simulink model "Vehicle_Motion_Model_R2014a"  (R2014a)
settings: Solver=ode4  SolverMode=SingleTasking  StartTime=0.0  StopTime=10.0  FixedStep=0.001  RelTol=1e-3
values from neighbouring files (symbols this model uses):
  chassis_real = chassis    [Parameters_Chassis.m]
  mu = [1 1 1 1]    [Parameters_Initialization.m]
  psi0 = 0    [Parameters_Initialization.m]
  psip0 = 0    [Parameters_Initialization.m]
  vx0 = 15    [Parameters_Initialization.m]
  vy0 = 0    [Parameters_Initialization.m]
  x0 = 0    [Parameters_Initialization.m]
  y0 = 0    [Parameters_Initialization.m]
undefined symbols (not defined in the file or in its folder): DiscIntNeverNeededParam, tireparam
libraries: vrlib x6, simulink x2
settings Model: CovMetricSettings=dwe  CovHtmlReporting=off  covSaveCumulativeToWorkspaceVar=off  CovSaveSingleToWorkspaceVar=off  CovExternalEMLEnable=on  CovSFcnEnable=on  Creator=Leo  LastModifiedBy=Leo
settings DataIOCC: LimitDataPoints=off  SaveFormat=StructureWithTime
settings DebuggingCC: MergeDetectMultiDrivingBlocksExec=error  SolverPrmCheckMsg=none  FrameProcessingCompatibilityMsg=error  SFUnexpectedBacktrackingDiag=error  SFNoUnconditionalDefaultTransitionDiag=error
settings HardwareCC: ProdBitPerPointer=64  ProdLargestAtomicFloat=Float  ProdIntDivRoundTo=Zero  ProdEndianess=LittleEndian  ProdHWDeviceType=Specified
settings ModelReferenceCC: PropagateSignalLabelsOutOfModel=on
settings GRTTargetCC: TargetLangStandard=C99 (ISO)  GeneratePreprocessorConditionals=Use local settings

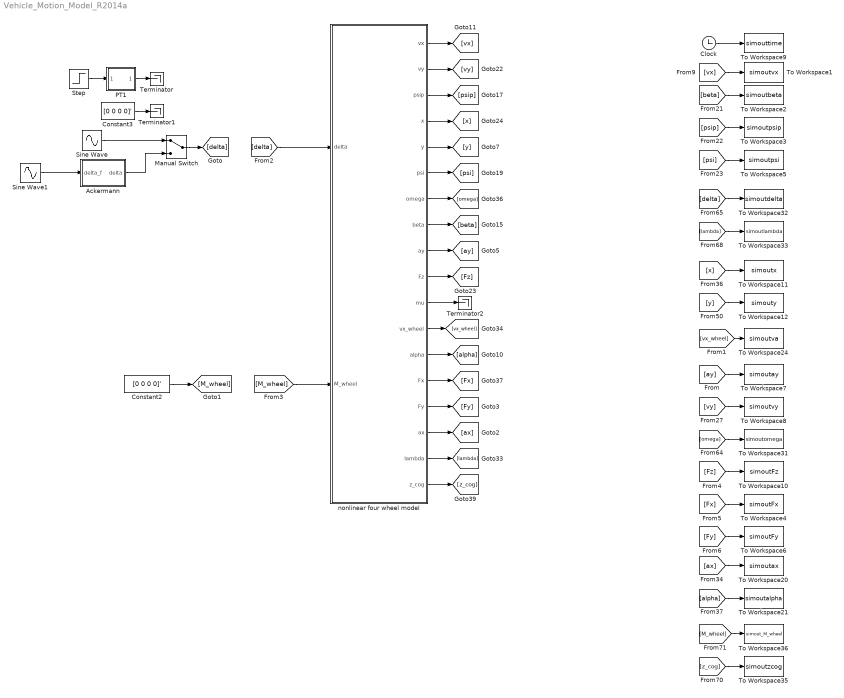
== system Vehicle_Motion_Model_R2014a ==
  Ackermann : Subsystem
  Clock : Clock
  Constant2 : Constant  Value=[0 0 0 0]'
  Constant3 : Constant  Value=[0 0 0 0]'
  Manual Switch : ManualSwitch
  PT1 : Subsystem
  Sine Wave : Sin  Amplitude=30/180*pi*[1 1 0 0]  Frequency=3  SampleTime=0
  Sine Wave1 : Sin  Amplitude=30/180*pi  Frequency=3  SampleTime=0
  Step : Step  Time=0.5  After=30/180*pi*[1 1 0 0]  SampleTime=0
  Terminator : Terminator
  Terminator1 : Terminator
  Terminator2 : Terminator
  To Workspace1 : ToWorkspace  VariableName=simoutvx  SaveFormat=Timeseries  SampleTime=-1
  To Workspace10 : ToWorkspace  VariableName=simoutFz  SaveFormat=Timeseries  SampleTime=-1
  To Workspace11 : ToWorkspace  VariableName=simoutx  SaveFormat=Timeseries  SampleTime=-1
  To Workspace12 : ToWorkspace  VariableName=simouty  SaveFormat=Timeseries  SampleTime=-1
  To Workspace2 : ToWorkspace  VariableName=simoutbeta  SaveFormat=Timeseries  SampleTime=-1
  To Workspace20 : ToWorkspace  VariableName=simoutax  SaveFormat=Timeseries  SampleTime=-1
  To Workspace21 : ToWorkspace  VariableName=simoutalpha  SaveFormat=Timeseries  SampleTime=-1
  To Workspace24 : ToWorkspace  VariableName=simoutva  SaveFormat=Timeseries  SampleTime=-1
  To Workspace3 : ToWorkspace  VariableName=simoutpsip  SaveFormat=Timeseries  SampleTime=-1
  To Workspace31 : ToWorkspace  VariableName=simoutomega  SaveFormat=Timeseries  SampleTime=-1
  To Workspace32 : ToWorkspace  VariableName=simoutdelta  SaveFormat=Timeseries  SampleTime=-1
  To Workspace33 : ToWorkspace  VariableName=simoutlambda  SaveFormat=Timeseries  SampleTime=-1
  To Workspace35 : ToWorkspace  VariableName=simoutzcog  SaveFormat=Timeseries  SampleTime=-1
  To Workspace36 : ToWorkspace  VariableName=simout_M_wheel  SaveFormat=Timeseries  SampleTime=-1
  To Workspace4 : ToWorkspace  VariableName=simoutFx  SaveFormat=Timeseries  SampleTime=-1
  To Workspace5 : ToWorkspace  VariableName=simoutpsi  SaveFormat=Timeseries  SampleTime=-1
  To Workspace6 : ToWorkspace  VariableName=simoutFy  SaveFormat=Timeseries  SampleTime=-1
  To Workspace7 : ToWorkspace  VariableName=simoutay  SaveFormat=Timeseries  SampleTime=-1
  To Workspace8 : ToWorkspace  VariableName=simoutvy  SaveFormat=Timeseries  SampleTime=-1
  To Workspace9 : ToWorkspace  VariableName=simouttime  SampleTime=-1
  nonlinear four wheel model : Subsystem  Description=|
      | vereinfachte alpha
      | beta=vs/vl
  wires:
  Step/1 -> PT1/1(In1)
  [delta] -> nonlinear four wheel model/1(delta)
  [lambda] -> To Workspace33/1
  [beta] -> To Workspace2/1
  [vx_wheel] -> To Workspace24/1
  nonlinear four wheel model/9(ay) -> [ay]
  [M_wheel] -> To Workspace36/1
  [z_cog] -> To Workspace35/1
  [delta] -> To Workspace32/1
  nonlinear four wheel model/10(Fz) -> [Fz]
  nonlinear four wheel model/12(vx_wheel) -> [vx_wheel]
  [y] -> To Workspace12/1
  [omega] -> To Workspace31/1
  [vy] -> To Workspace8/1
  [alpha] -> To Workspace21/1
  Clock/1 -> To Workspace9/1
  [ax] -> To Workspace20/1
  nonlinear four wheel model/14(Fx) -> [Fx]
  Sine Wave1/1 -> Ackermann/1(delta_f)
  [vx] -> To Workspace1/1
  [x] -> To Workspace11/1
  nonlinear four wheel model/6(psi) -> [psi]
  nonlinear four wheel model/16(ax) -> [ax]
  nonlinear four wheel model/5(y) -> [y]
  [psip] -> To Workspace3/1
  nonlinear four wheel model/7(omega) -> [omega]
  nonlinear four wheel model/11(mu) -> Terminator2/1
  nonlinear four wheel model/13(alpha) -> [alpha]
  nonlinear four wheel model/1(vx) -> [vx]
  nonlinear four wheel model/18(z_cog) -> [z_cog]
  [ay] -> To Workspace7/1
  nonlinear four wheel model/2(vy) -> [vy]
  [psi] -> To Workspace5/1
  nonlinear four wheel model/3(psip) -> [psip]
  nonlinear four wheel model/17(lambda) -> [lambda]
  [M_wheel] -> nonlinear four wheel model/2(M_wheel)
  nonlinear four wheel model/4(x) -> [x]
  nonlinear four wheel model/8(beta) -> [beta]
  Sine Wave/1 -> Manual Switch/1
  Ackermann/1(delta) -> Manual Switch/2
  PT1/1(Out1) -> Terminator/1
  Constant3/1 -> Terminator1/1
  Manual Switch/1 -> [delta]
  Constant2/1 -> [M_wheel]
  [Fy] -> To Workspace6/1
  [Fx] -> To Workspace4/1
  [Fz] -> To Workspace10/1
  nonlinear four wheel model/15(Fy) -> [Fy]

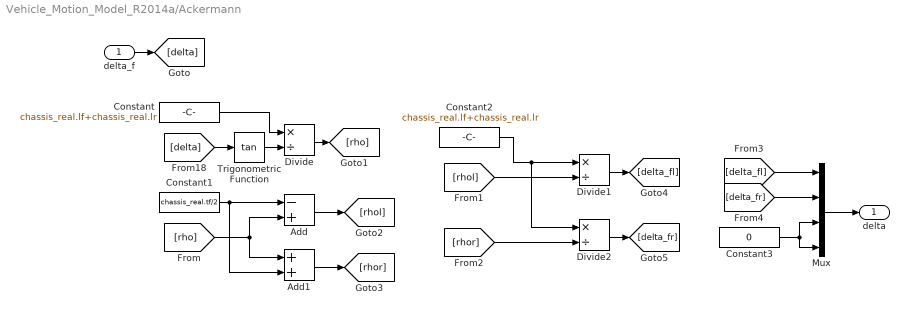
== system Vehicle_Motion_Model_R2014a/Ackermann ==
  delta_f : Inport
  Add : Sum  Inputs=-+
  Add1 : Sum
  Constant : Constant  Value=chassis_real.lf+chassis_real.lr
  Constant1 : Constant  Value=chassis_real.tf/2
  Constant2 : Constant  Value=chassis_real.lf+chassis_real.lr
  Constant3 : Constant  Value=0
  Divide : Product  Inputs=*/
  Divide1 : Product  Inputs=*/
  Divide2 : Product  Inputs=*/
  Mux : Mux
  Trigonometric Function : Trigonometry  Operator=tan
  delta : Outport
  wires:
  delta_f/1 -> [delta]
  [delta] -> Trigonometric Function/1
  Trigonometric Function/1 -> Divide/2
  Constant/1 -> Divide/1
  Divide/1 -> [rho]
  Add/1 -> [rhol]
  [rho] -> Add/2, Add1/1
  Constant1/1 -> Add1/2, Add/1
  Add1/1 -> [rhor]
  Constant2/1 -> Divide2/1, Divide1/1
  [rhol] -> Divide1/2
  [rhor] -> Divide2/2
  Divide1/1 -> [delta_fl]
  Divide2/1 -> [delta_fr]
  Mux/1 -> delta/1
  [delta_fl] -> Mux/1
  [delta_fr] -> Mux/2
  Constant3/1 -> Mux/4, Mux/3

== system Vehicle_Motion_Model_R2014a/PT1 ==
  In1 : Inport
  Add : Sum  Inputs=+-
  Gain : Gain
  Integrator : Integrator
  Out1 : Outport
  wires:
  Add/1 -> Integrator/1
  Integrator/1 -> Gain/1
  Gain/1 -> Add/2, Out1/1
  In1/1 -> Add/1

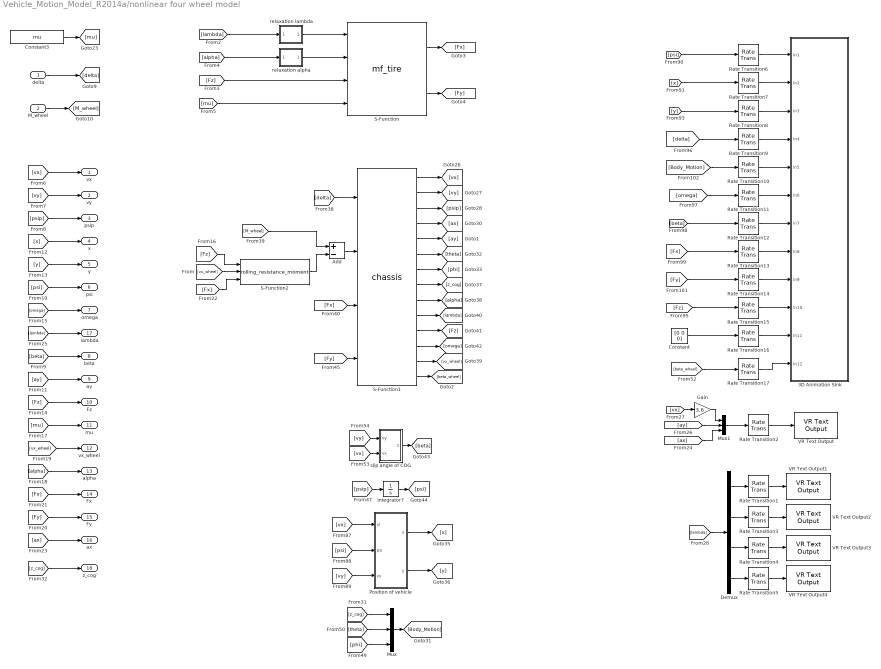
== system Vehicle_Motion_Model_R2014a/nonlinear four wheel model ==
  delta : Inport
  M_wheel : Inport  Port=2
  3D Animation Sink : Subsystem
  Add : Sum  Inputs=+-
  Constant : Constant  Value=[0 0 0]
  Constant3 : Constant  Value=mu
  Demux : Demux
  Gain : Gain  Gain=3.6
  Integrator7 : Integrator  InitialCondition=psi0
  Mux : Mux  Inputs=3
  Mux1 : Mux  Inputs=3
  Position of vehicle : Subsystem
  Rate Transition{1..17} (17 alike) : RateTransition  Integrity=off
  S-Function : S-Function  FunctionName=mf_tire  Parameters=tireparam.ov,tireparam.fxp,tireparam.fyp,tireparam.fxc,tireparam.fyc  SFunctionDeploymentMode=off  EnableBusSupport=off
  S-Function1 : S-Function  FunctionName=chassis  Parameters=chassis_real.lf,chassis_real.lr,chassis_real.tf,chassis_real.tr,chassis_real.m,chassis_real.jz,chassis_real.jy,chassis_real.jx,chassis_real.h,chassis_real.df,chassis_real.dr,chassis_real.kf,chassis_real.kr,chassis_real.jwheel,chassis_real.rwheel,vx0,vy0,psip0  SFunctionDeploymentMode=off  EnableBusSupport=off
  S-Function2 : S-Function  FunctionName=rolling_resistance_moment  Parameters=tireparam.ov,tireparam.mroll  SFunctionDeploymentMode=off  EnableBusSupport=off
  VR Text Output : vrlib/VR Text Output  VrmlFile=Virtual World Vehicle.wrl  TxtNode=lefttop  FormatString="Speed  :  %3.1f km/h \\nay        :  %1.1f g \\nax        :  %1.1f g"  Ts=0.01  ForceViewerOpen=off
  VR Text Output1 : vrlib/VR Text Output  VrmlFile=Virtual World Vehicle.wrl  TxtNode=lft  FormatString=%1.2f  Ts=0.01  ForceViewerOpen=off
  VR Text Output2 : vrlib/VR Text Output  VrmlFile=Virtual World Vehicle.wrl  TxtNode=rft  FormatString=%1.2f  Ts=0.01  ForceViewerOpen=off
  VR Text Output3 : vrlib/VR Text Output  VrmlFile=Virtual World Vehicle.wrl  TxtNode=lrt  FormatString=%1.2f  Ts=0.01  ForceViewerOpen=off
  VR Text Output4 : vrlib/VR Text Output  VrmlFile=Virtual World Vehicle.wrl  TxtNode=rrt  FormatString=%1.2f  Ts=0.01  ForceViewerOpen=off
  relaxation alpha : Subsystem
  relaxation lambda : Subsystem
  slip angle of COG : Subsystem
  vx : Outport
  vy : Outport  Port=2
  psip : Outport  Port=3
  x : Outport  Port=4
  y : Outport  Port=5
  psi : Outport  Port=6
  omega : Outport  Port=7
  beta : Outport  Port=8
  ay : Outport  Port=9
  Fz : Outport  Port=10
  mu : Outport  Port=11
  vx_wheel : Outport  Port=12
  alpha : Outport  Port=13
  Fx : Outport  Port=14
  Fy : Outport  Port=15
  ax : Outport  Port=16
  lambda : Outport  Port=17
  z_cog : Outport  Port=18
  wires:
  Constant3/1 -> [mu]
  [vx] -> Position of vehicle/1(vl)
  [psi] -> Position of vehicle/2(psi)
  [vy] -> Position of vehicle/3(vs)
  Position of vehicle/1(x) -> [x]
  Position of vehicle/2(y) -> [y]
  delta/1 -> [delta]
  [vx] -> vx/1
  [vy] -> vy/1
  [psip] -> psip/1
  [psi] -> psi/1
  [ay] -> ay/1
  [beta] -> beta/1
  [x] -> x/1
  [y] -> y/1
  [omega] -> omega/1
  [Fz] -> Fz/1
  [mu] -> mu/1
  [vx_wheel] -> vx_wheel/1
  [alpha] -> alpha/1
  [Fx] -> Fx/1
  [Fy] -> Fy/1
  [ax] -> ax/1
  [lambda] -> lambda/1
  [z_cog] -> z_cog/1
  [omega] -> Rate Transition11/1
  [delta] -> Rate Transition9/1
  [psi] -> Rate Transition6/1
  [x] -> Rate Transition7/1
  [beta] -> Rate Transition12/1
  [Fx] -> Rate Transition13/1
  [Body_Motion] -> Rate Transition10/1
  [Fy] -> Rate Transition14/1
  [y] -> Rate Transition8/1
  [Fz] -> Rate Transition15/1
  Mux/1 -> [Body_Motion]
  [phi] -> Mux/3
  [theta] -> Mux/2
  [z_cog] -> Mux/1
  Mux1/1 -> Rate Transition2/1
  [ay] -> Mux1/2
  [vx] -> Gain/1
  [ax] -> Mux1/3
  Rate Transition2/1 -> VR Text Output/1
  Rate Transition1/1 -> VR Text Output1/1
  Demux/1 -> Rate Transition1/1
  [lambda] -> Demux/1
  Rate Transition3/1 -> VR Text Output2/1
  Demux/2 -> Rate Transition3/1
  Rate Transition4/1 -> VR Text Output3/1
  Demux/3 -> Rate Transition4/1
  Rate Transition5/1 -> VR Text Output4/1
  Demux/4 -> Rate Transition5/1
  Rate Transition6/1 -> 3D Animation Sink/1(In1)
  Rate Transition7/1 -> 3D Animation Sink/2(In2)
  Rate Transition8/1 -> 3D Animation Sink/3(In3)
  Rate Transition9/1 -> 3D Animation Sink/4(In4)
  Rate Transition10/1 -> 3D Animation Sink/5(In5)
  Rate Transition11/1 -> 3D Animation Sink/6(In6)
  Rate Transition12/1 -> 3D Animation Sink/7(In7)
  Rate Transition13/1 -> 3D Animation Sink/8(In8)
  Rate Transition14/1 -> 3D Animation Sink/9(In9)
  Rate Transition15/1 -> 3D Animation Sink/10(In10)
  Gain/1 -> Mux1/1
  M_wheel/1 -> [M_wheel]
  Integrator7/1 -> [psi]
  S-Function1/7 -> [phi]
  [psip] -> Integrator7/1
  [delta] -> S-Function1/1
  S-Function1/8 -> [z_cog]
  S-Function1/5 -> [ay]
  S-Function1/4 -> [ax]
  S-Function1/1 -> [vx]
  S-Function1/11 -> [Fz]
  [Fx] -> S-Function1/3
  [Fy] -> S-Function1/4
  S-Function1/3 -> [psip]
  S-Function1/12 -> [omega]
  [M_wheel] -> Add/1
  S-Function1/10 -> [lambda]
  S-Function1/2 -> [vy]
  S-Function1/6 -> [theta]
  S-Function1/9 -> [alpha]
  S-Function1/13 -> [vx_wheel]
  Rate Transition17/1 -> 3D Animation Sink/12(In12)
  [beta_wheel] -> Rate Transition17/1
  [mu] -> S-Function/4
  [lambda] -> relaxation lambda/1(In1)
  [Fz] -> S-Function/3
  S-Function/1 -> [Fx]
  S-Function/2 -> [Fy]
  [alpha] -> relaxation alpha/1(In1)
  relaxation lambda/1(Out1) -> S-Function/1
  relaxation alpha/1(Out1) -> S-Function/2
  [vy] -> slip angle of COG/1(vy)
  [vx] -> slip angle of COG/2(vx)
  slip angle of COG/1(beta) -> [beta]
  Add/1 -> S-Function1/2
  [vx_wheel] -> S-Function2/2
  [Fz] -> S-Function2/1
  [Fx] -> S-Function2/3
  S-Function1/14 -> [beta_wheel]
  S-Function2/1 -> Add/2
  Rate Transition16/1 -> 3D Animation Sink/11(In11)
  Constant/1 -> Rate Transition16/1

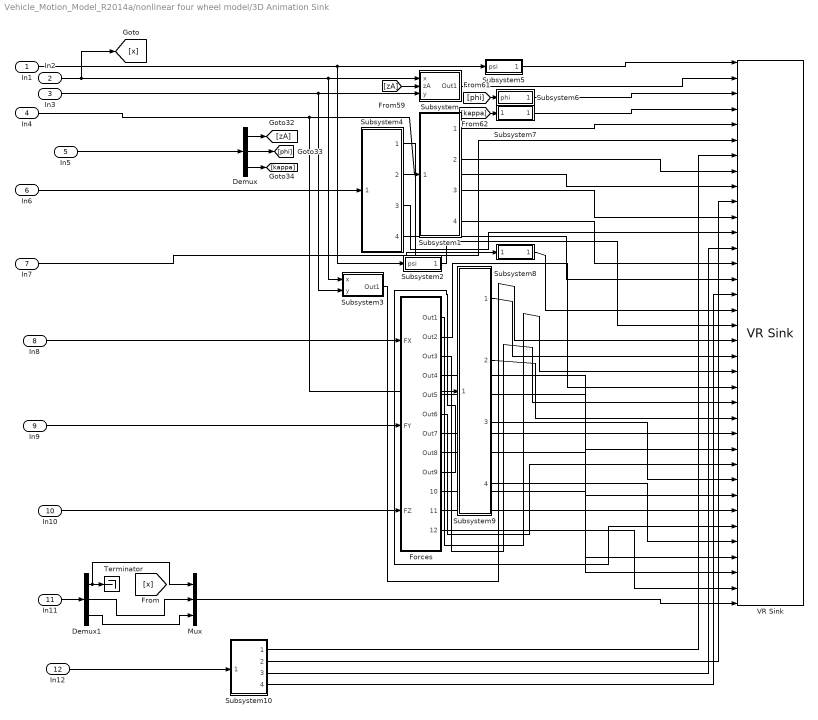
== system Vehicle_Motion_Model_R2014a/nonlinear four wheel model/3D Animation Sink ==
  In1 : Inport
  In2 : Inport  Port=2
  In3 : Inport  Port=3
  In4 : Inport  Port=4
  In5 : Inport  Port=5
  In6 : Inport  Port=6
  In7 : Inport  Port=7
  In8 : Inport  Port=8
  In9 : Inport  Port=9
  In10 : Inport  Port=10
  In11 : Inport  Port=11
  In12 : Inport  Port=12
  Demux : Demux  Outputs=3
  Demux1 : Demux  Outputs=3
  Forces : Subsystem
  Mux : Mux  Inputs=3
  Subsystem : Subsystem
  Subsystem1 : Subsystem
  Subsystem10 : Subsystem
  Subsystem2 : Subsystem
  Subsystem3 : Subsystem
  Subsystem4 : Subsystem
  Subsystem5 : Subsystem
  Subsystem6 : Subsystem
  Subsystem7 : Subsystem
  Subsystem8 : Subsystem
  Subsystem9 : Subsystem
  Terminator : Terminator
  VR Sink : vrlib/VR Sink  InstantiateOnLoad=on  SampleTime=0.02  ViewEnable=on  RemoteChange=off  RemoteView=off  FieldsWritten=Carbody.rotation.4.1.1.double#Carbody.translation.3.1.1.double#Nicken.rotation.4.1.1.double#carbody.rotation.4.1.1.double#SLF.rotation.4.1.1.double#TyreLF.rotation.4.1.1.double#VLF.rotation.4.1.1.double#SRF.rotation.4.1.1.double#TyreRF.rotation.4.1.1.double#VRF.rotation.4.1.1.double#SLR.rotation.4.1.1.double#TyreLR.rotation.4.1.1.double#VLR.rotation.4.1.1.double#SRR.rotation.4.1.1.double#TyreRR.rotation.4.1.1.double#VRR.rotation.4.1.1.double#Vcar.rotation.4.1.1.double#Position2D.rotation.4.1.1.double#Position2D.translation.3.1.1.double#LFforce.rotation.4.1.1.double#LFblue.scale.3.1.1.double#LFred.scale.3.1.1.double#LFgreen.scale.3.1.1.double#RFforce.rotation.4.1.1.double#RFblue.scale.3.1.1.double#RFred.scale.3.1.1.double#RFgreen.scale.3.1.1.double#LRforce.rotation.4.1.1.double#LRblue.scale.3.1.1.double#LRred.scale.3.1.1.double#LRgreen.scale.3.1.1.double#RRforce.rotation.4.1.1.double#RRblue.scale.3.1.1.double#RRred.scale.3.1.1.double#RRgreen.scale.3.1.1.double#PositionTrajectory.translation.3.1.1.double  WorldFileName=Virtual World Vehicle.wrl  AutoView=off  VideoDimensions=[]  AllowVariableSize=off
  wires:
  In4/1 -> Subsystem9/1(DELTA), Subsystem1/1(DELTA)
  Demux/2 -> [phi]
  [phi] -> Subsystem6/1(phi)
  [kappa] -> Subsystem7/1(kappa)
  In8/1 -> Forces/1(FX)
  [zA] -> Subsystem/2(zA)
  In9/1 -> Forces/2(FY)
  In3/1 -> Subsystem3/2(y), Subsystem/3(y)
  In7/1 -> Subsystem8/1(beta)
  In2/1 -> [x], Subsystem3/1(x), Subsystem/1(x)
  In5/1 -> Demux/1
  Demux/1 -> [zA]
  Demux/3 -> [kappa]
  In6/1 -> Subsystem4/1(OMEGA)
  In10/1 -> Forces/3(FZ)
  In1/1 -> Subsystem2/1(psi), Subsystem5/1(psi)
  In11/1 -> Demux1/1
  Demux1/1 -> Mux/1, Terminator/1
  Demux1/2 -> Mux/2
  Demux1/3 -> Mux/3
  Subsystem5/1(Out1) -> VR Sink/1
  Subsystem/1(Out1) -> VR Sink/2
  Subsystem6/1(Out1) -> VR Sink/3
  Subsystem7/1(Out1) -> VR Sink/4
  Subsystem1/1(Out1) -> VR Sink/5
  Subsystem4/1(Out1) -> VR Sink/6
  Subsystem1/2(Out2) -> VR Sink/8
  Subsystem4/2(Out2) -> VR Sink/9
  Subsystem1/3(Out3) -> VR Sink/11
  Subsystem4/3(Out3) -> VR Sink/12
  Subsystem1/4(Out4) -> VR Sink/14
  Subsystem4/4(Out4) -> VR Sink/15
  Subsystem8/1(Out1) -> VR Sink/17
  Subsystem2/1(Out1) -> VR Sink/18
  Subsystem3/1(Out1) -> VR Sink/19
  Subsystem9/1(Out1) -> VR Sink/20
  Forces/1(Out1) -> VR Sink/21
  Forces/2(Out2) -> VR Sink/22
  Forces/3(Out3) -> VR Sink/23
  Subsystem9/2(Out2) -> VR Sink/24
  Forces/4(Out4) -> VR Sink/25
  Forces/5(Out5) -> VR Sink/26
  Forces/6(Out6) -> VR Sink/27
  Subsystem9/3(Out3) -> VR Sink/28
  Forces/7(Out7) -> VR Sink/29
  Forces/8(Out8) -> VR Sink/30
  Forces/9(Out9) -> VR Sink/31
  Subsystem9/4(Out4) -> VR Sink/32
  Forces/10(Out10) -> VR Sink/33
  Forces/11(Out11) -> VR Sink/34
  Forces/12(Out12) -> VR Sink/35
  Mux/1 -> VR Sink/36
  In12/1 -> Subsystem10/1(VRad)
  Subsystem10/2(Out2) -> VR Sink/10
  Subsystem10/3(Out3) -> VR Sink/13
  Subsystem10/4(Out4) -> VR Sink/16
  Subsystem10/1(Out1) -> VR Sink/7

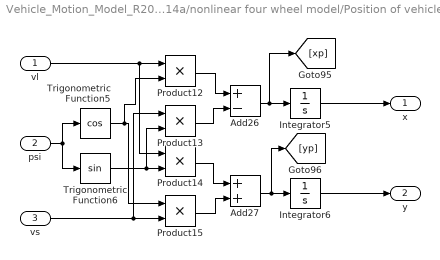
== system Vehicle_Motion_Model_R2014a/nonlinear four wheel model/Position of vehicle ==
  vl : Inport
  psi : Inport  Port=2
  vs : Inport  Port=3
  Add26 : Sum  Inputs=+-
  Add27 : Sum
  Integrator5 : Integrator  InitialCondition=x0
  Integrator6 : Integrator  InitialCondition=y0
  Product{12..15} (4 alike) : Product
  Trigonometric Function5 : Trigonometry  Operator=cos
  Trigonometric Function6 : Trigonometry
  x : Outport
  y : Outport  Port=2
  wires:
  Product15/1 -> Add27/2
  Product13/1 -> Add26/2
  Add27/1 -> [yp], Integrator6/1
  vl/1 -> Product14/1, Product12/1
  Product14/1 -> Add27/1
  Trigonometric Function5/1 -> Product15/1, Product12/2
  Trigonometric Function6/1 -> Product14/2, Product13/2
  Integrator5/1 -> x/1
  Product12/1 -> Add26/1
  Add26/1 -> [xp], Integrator5/1
  psi/1 -> Trigonometric Function5/1, Trigonometric Function6/1
  vs/1 -> Product15/2, Product13/1
  Integrator6/1 -> y/1

== system Vehicle_Motion_Model_R2014a/nonlinear four wheel model/relaxation alpha ==
  In1 : Inport
  Add : Sum  Inputs=+-
  Gain : Gain  Gain=100
  Integrator : Integrator
  Out1 : Outport
  wires:
  In1/1 -> Add/1
  Gain/1 -> Out1/1, Add/2
  Integrator/1 -> Gain/1
  Add/1 -> Integrator/1

== system Vehicle_Motion_Model_R2014a/nonlinear four wheel model/relaxation lambda ==
  In1 : Inport
  Add : Sum  Inputs=+-
  Gain : Gain  Gain=100
  Integrator : Integrator
  Out1 : Outport
  wires:
  Add/1 -> Integrator/1
  Integrator/1 -> Gain/1
  Gain/1 -> Add/2, Out1/1
  In1/1 -> Add/1

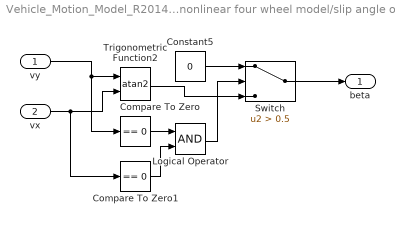
== system Vehicle_Motion_Model_R2014a/nonlinear four wheel model/slip angle of COG ==
  vy : Inport
  vx : Inport  Port=2
  Compare To Zero : simulink/Logic and Bit Operations/Compare To Zero  relop===  OutDataTypeStr=boolean
  Compare To Zero1 : simulink/Logic and Bit Operations/Compare To Zero  relop===  OutDataTypeStr=boolean
  Constant5 : Constant  Value=0
  Logical Operator : Logic  AllPortsSameDT=off  OutDataTypeStr=boolean
  Switch : Switch  Criteria=u2 > Threshold  Threshold=0.5
  Trigonometric Function2 : Trigonometry  Operator=atan2
  beta : Outport
  wires:
  Constant5/1 -> Switch/1
  vx/1 -> Compare To Zero1/1, Trigonometric Function2/2
  Compare To Zero1/1 -> Logical Operator/2
  Switch/1 -> beta/1
  Logical Operator/1 -> Switch/2
  Compare To Zero/1 -> Logical Operator/1
  Trigonometric Function2/1 -> Switch/3
  vy/1 -> Compare To Zero/1, Trigonometric Function2/1

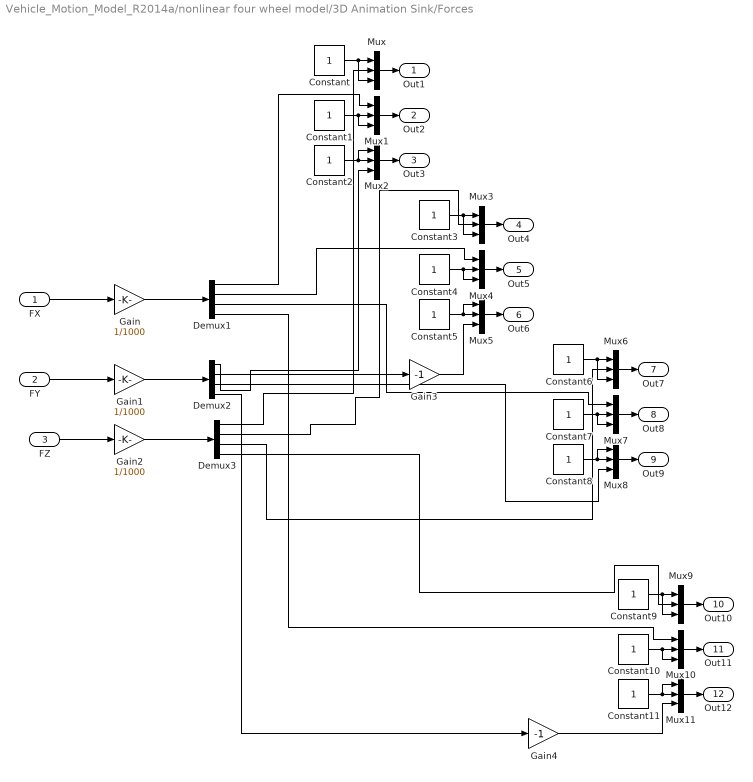
== system Vehicle_Motion_Model_R2014a/nonlinear four wheel model/3D Animation Sink/Forces ==
  FX : Inport
  FY : Inport  Port=2
  FZ : Inport  Port=3
  Constant{,1..11} (12 alike) : Constant
  Demux1 : Demux
  Demux2 : Demux
  Demux3 : Demux
  Gain : Gain  Gain=1/1000
  Gain1 : Gain  Gain=1/1000
  Gain2 : Gain  Gain=1/1000
  Gain3 : Gain  Gain=-1
  Gain4 : Gain  Gain=-1
  Mux{,1..11} (12 alike) : Mux  Inputs=3
  Out1 : Outport
  Out2 : Outport  Port=2
  Out3 : Outport  Port=3
  Out4 : Outport  Port=4
  Out5 : Outport  Port=5
  Out6 : Outport  Port=6
  Out7 : Outport  Port=7
  Out8 : Outport  Port=8
  Out9 : Outport  Port=9
  Out10 : Outport  Port=10
  Out11 : Outport  Port=11
  Out12 : Outport  Port=12
  wires:
  FZ/1 -> Gain2/1
  FX/1 -> Gain/1
  Demux1/1 -> Mux1/1
  Demux3/1 -> Mux/2
  Mux/1 -> Out1/1
  FY/1 -> Gain1/1
  Gain/1 -> Demux1/1
  Gain1/1 -> Demux2/1
  Gain2/1 -> Demux3/1
  Constant/1 -> Mux/3, Mux/1
  Mux1/1 -> Out2/1
  Constant1/1 -> Mux1/2, Mux1/3
  Demux2/1 -> Mux2/3
  Mux2/1 -> Out3/1
  Constant2/1 -> Mux2/1, Mux2/2
  Demux1/2 -> Mux4/1
  Mux3/1 -> Out4/1
  Constant3/1 -> Mux3/1, Mux3/3
  Mux4/1 -> Out5/1
  Constant4/1 -> Mux4/3, Mux4/2
  Demux3/2 -> Mux3/2
  Mux5/1 -> Out6/1
  Constant5/1 -> Mux5/2, Mux5/1
  Demux1/3 -> Mux7/1
  Demux3/3 -> Mux6/2
  Mux6/1 -> Out7/1
  Constant6/1 -> Mux6/3, Mux6/1
  Mux7/1 -> Out8/1
  Constant7/1 -> Mux7/2, Mux7/3
  Demux2/3 -> Mux8/3
  Mux8/1 -> Out9/1
  Constant8/1 -> Mux8/1, Mux8/2
  Demux1/4 -> Mux10/1
  Mux9/1 -> Out10/1
  Constant9/1 -> Mux9/1, Mux9/3
  Mux10/1 -> Out11/1
  Constant10/1 -> Mux10/3, Mux10/2
  Demux3/4 -> Mux9/2
  Mux11/1 -> Out12/1
  Constant11/1 -> Mux11/2, Mux11/1
  Demux2/2 -> Gain3/1
  Demux2/4 -> Gain4/1
  Gain3/1 -> Mux5/3
  Gain4/1 -> Mux11/3

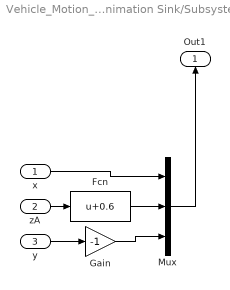
== system Vehicle_Motion_Model_R2014a/nonlinear four wheel model/3D Animation Sink/Subsystem ==
  x : Inport
  zA : Inport  Port=2
  y : Inport  Port=3
  Fcn : Fcn  Expr=u+0.6
  Gain : Gain  Gain=-1
  Mux : Mux  Inputs=3
  Out1 : Outport
  wires:
  zA/1 -> Fcn/1
  x/1 -> Mux/1
  y/1 -> Gain/1
  Mux/1 -> Out1/1
  Gain/1 -> Mux/3
  Fcn/1 -> Mux/2

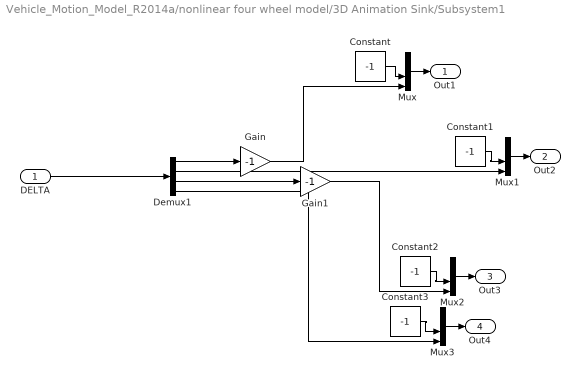
== system Vehicle_Motion_Model_R2014a/nonlinear four wheel model/3D Animation Sink/Subsystem1 ==
  DELTA : Inport
  Constant{,1..3} (4 alike) : Constant  Value=-1
  Demux1 : Demux
  Gain : Gain  Gain=-1
  Gain1 : Gain  Gain=-1
  Mux{,1..3} (4 alike) : Mux
  Out1 : Outport
  Out2 : Outport  Port=2
  Out3 : Outport  Port=3
  Out4 : Outport  Port=4
  wires:
  DELTA/1 -> Demux1/1
  Constant3/1 -> Mux3/3
  Mux3/1 -> Out4/1
  Constant2/1 -> Mux2/3
  Mux2/1 -> Out3/1
  Constant1/1 -> Mux1/3
  Mux1/1 -> Out2/1
  Constant/1 -> Mux/3
  Mux/1 -> Out1/1
  Demux1/4 -> Mux3/4
  Demux1/1 -> Gain/1
  Demux1/3 -> Gain1/1
  Demux1/2 -> Mux1/4
  Gain/1 -> Mux/4
  Gain1/1 -> Mux2/4

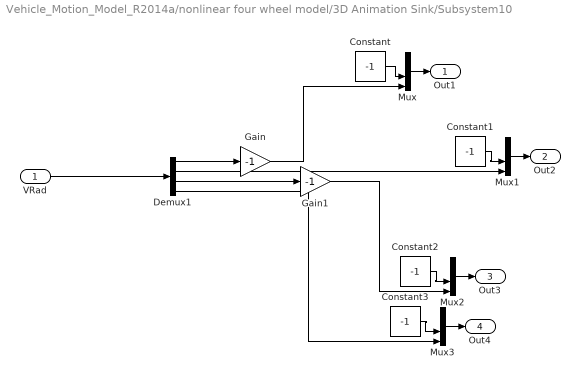
== system Vehicle_Motion_Model_R2014a/nonlinear four wheel model/3D Animation Sink/Subsystem10 ==
  VRad : Inport
  Constant{,1..3} (4 alike) : Constant  Value=-1
  Demux1 : Demux
  Gain : Gain  Gain=-1
  Gain1 : Gain  Gain=-1
  Mux{,1..3} (4 alike) : Mux
  Out1 : Outport
  Out2 : Outport  Port=2
  Out3 : Outport  Port=3
  Out4 : Outport  Port=4
  wires:
  VRad/1 -> Demux1/1
  Constant3/1 -> Mux3/3
  Mux3/1 -> Out4/1
  Constant2/1 -> Mux2/3
  Mux2/1 -> Out3/1
  Constant1/1 -> Mux1/3
  Mux1/1 -> Out2/1
  Constant/1 -> Mux/3
  Mux/1 -> Out1/1
  Demux1/4 -> Mux3/4
  Demux1/1 -> Gain/1
  Demux1/3 -> Gain1/1
  Demux1/2 -> Mux1/4
  Gain/1 -> Mux/4
  Gain1/1 -> Mux2/4

== system Vehicle_Motion_Model_R2014a/nonlinear four wheel model/3D Animation Sink/Subsystem2 ==
  psi : Inport
  Constant : Constant
  Constant1 : Constant  Value=0
  Mux1 : Mux
  Out1 : Outport
  wires:
  Mux1/1 -> Out1/1
  Constant1/1 -> Mux1/1, Mux1/3
  Constant/1 -> Mux1/2
  psi/1 -> Mux1/4

== system Vehicle_Motion_Model_R2014a/nonlinear four wheel model/3D Animation Sink/Subsystem3 ==
  x : Inport
  y : Inport  Port=2
  Gain : Gain  Gain=-1
  Mux : Mux  Inputs=3
  Out1 : Outport
  wires:
  x/1 -> Mux/1
  y/1 -> Gain/1
  Mux/1 -> Out1/1
  Gain/1 -> Mux/3

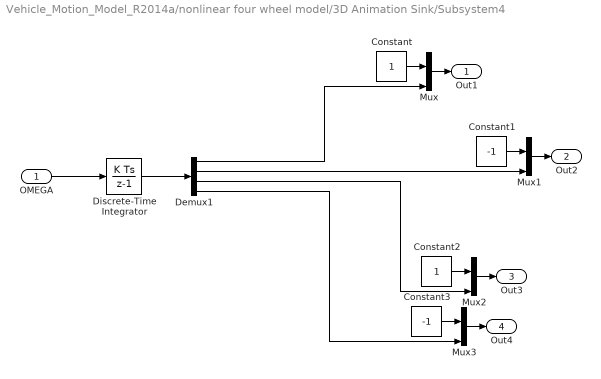
== system Vehicle_Motion_Model_R2014a/nonlinear four wheel model/3D Animation Sink/Subsystem4 ==
  OMEGA : Inport
  Constant : Constant
  Constant1 : Constant  Value=-1
  Constant2 : Constant
  Constant3 : Constant  Value=-1
  Demux1 : Demux
  Discrete-Time Integrator : DiscreteIntegrator  InitialConditionSetting=State (most efficient)  SampleTime=-1  ICPrevOutput=DiscIntNeverNeededParam  ICPrevScaledInput=DiscIntNeverNeededParam
  Mux{,1..3} (4 alike) : Mux
  Out1 : Outport
  Out2 : Outport  Port=2
  Out3 : Outport  Port=3
  Out4 : Outport  Port=4
  wires:
  Demux1/2 -> Mux1/4
  Demux1/3 -> Mux2/4
  Demux1/1 -> Mux/4
  Demux1/4 -> Mux3/4
  OMEGA/1 -> Discrete-Time Integrator/1
  Mux/1 -> Out1/1
  Constant/1 -> Mux/2
  Mux1/1 -> Out2/1
  Constant1/1 -> Mux1/2
  Mux2/1 -> Out3/1
  Constant2/1 -> Mux2/2
  Mux3/1 -> Out4/1
  Constant3/1 -> Mux3/2
  Discrete-Time Integrator/1 -> Demux1/1

== system Vehicle_Motion_Model_R2014a/nonlinear four wheel model/3D Animation Sink/Subsystem5 ==
  psi : Inport
  Constant : Constant
  Constant1 : Constant  Value=0
  Mux1 : Mux
  Out1 : Outport
  wires:
  psi/1 -> Mux1/4
  Constant/1 -> Mux1/2
  Constant1/1 -> Mux1/3, Mux1/1
  Mux1/1 -> Out1/1

== system Vehicle_Motion_Model_R2014a/nonlinear four wheel model/3D Animation Sink/Subsystem6 ==
  phi : Inport
  Constant : Constant  Value=-1
  Constant1 : Constant  Value=0
  Mux1 : Mux
  Out1 : Outport
  wires:
  phi/1 -> Mux1/4
  Constant/1 -> Mux1/3
  Constant1/1 -> Mux1/2, Mux1/1
  Mux1/1 -> Out1/1

== system Vehicle_Motion_Model_R2014a/nonlinear four wheel model/3D Animation Sink/Subsystem7 ==
  kappa : Inport
  Constant : Constant
  Constant1 : Constant  Value=0
  Mux1 : Mux
  Out1 : Outport
  wires:
  Mux1/1 -> Out1/1
  Constant1/1 -> Mux1/3, Mux1/2
  Constant/1 -> Mux1/1
  kappa/1 -> Mux1/4

== system Vehicle_Motion_Model_R2014a/nonlinear four wheel model/3D Animation Sink/Subsystem8 ==
  beta : Inport
  Constant : Constant
  Constant1 : Constant  Value=0
  Mux1 : Mux
  Out1 : Outport
  wires:
  Mux1/1 -> Out1/1
  Constant1/1 -> Mux1/1, Mux1/3
  Constant/1 -> Mux1/2
  beta/1 -> Mux1/4

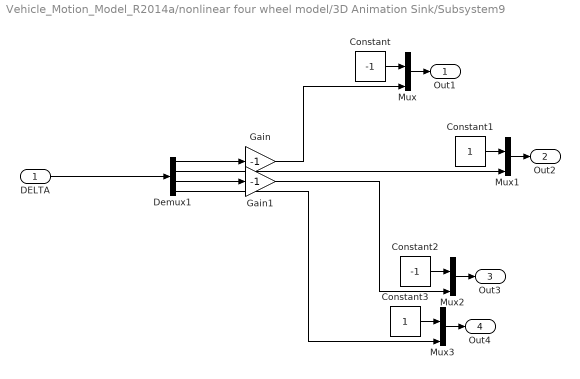
== system Vehicle_Motion_Model_R2014a/nonlinear four wheel model/3D Animation Sink/Subsystem9 ==
  DELTA : Inport
  Constant : Constant  Value=-1
  Constant1 : Constant
  Constant2 : Constant  Value=-1
  Constant3 : Constant
  Demux1 : Demux
  Gain : Gain  Gain=-1
  Gain1 : Gain  Gain=-1
  Mux{,1..3} (4 alike) : Mux
  Out1 : Outport
  Out2 : Outport  Port=2
  Out3 : Outport  Port=3
  Out4 : Outport  Port=4
  wires:
  Demux1/2 -> Mux1/4
  Demux1/3 -> Gain1/1
  Demux1/1 -> Gain/1
  Demux1/4 -> Mux3/4
  Mux/1 -> Out1/1
  Constant/1 -> Mux/2
  Mux1/1 -> Out2/1
  Constant1/1 -> Mux1/2
  Mux2/1 -> Out3/1
  Constant2/1 -> Mux2/2
  Mux3/1 -> Out4/1
  Constant3/1 -> Mux3/2
  DELTA/1 -> Demux1/1
  Gain/1 -> Mux/4
  Gain1/1 -> Mux2/4
